simulink model "feedback_hall_sensor"  (R2015a)
settings: Solver=ode45  StartTime=0.0  StopTime=2  RelTol=1e-3
values from neighbouring files (symbols this model uses):
  s = tf('s')    [delay.m]    (also in hall_effect_assign3.m; hall_effect_assign4.m; rhp_zero.m; rhp_zero_disturbance_vi.m)
libraries: cstblocks x2
settings Model: Creator=Kripa95  LastModifiedBy=Kripa95

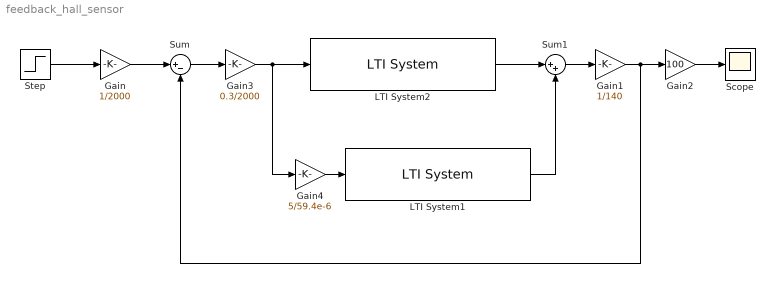
== system feedback_hall_sensor ==
  Gain : Gain  Gain=1/2000
  Gain1 : Gain  Gain=1/140
  Gain2 : Gain  Gain=100
  Gain3 : Gain  Gain=0.3/2000
  Gain4 : Gain  Gain=5/59.4e-6
  LTI System1 : cstblocks/LTI System  sys=((s+3.04e5)*(s-2.83e5))/(s*(s+20000))  IC=[]
  LTI System2 : cstblocks/LTI System  sys=2000*s/(s+100000)  IC=[]
  Scope : Scope
      settings: TimeRange=2  YMin=-1.445e+07  YMax=-1.3875e+07
  Step : Step  SampleTime=0
  Sum : Sum  Inputs=|+-
  Sum1 : Sum  Inputs=|++
  wires:
  Gain/1 -> Sum/1
  Gain2/1 -> Scope/1
  Step/1 -> Gain/1
  Gain4/1 -> LTI System1/1
  LTI System1/1 -> Sum1/2
  Sum1/1 -> Gain1/1
  Gain1/1 -> Sum/2, Gain2/1
  Gain3/1 -> LTI System2/1, Gain4/1
  Sum/1 -> Gain3/1
  LTI System2/1 -> Sum1/1
